simulink model "MotorControl_4"  (Simulink 8.1)
settings: Solver=FixedStepDiscrete  StartTime=0.0  StopTime=20  FixedStep=0.02  RelTol=1e-3
PostLoadFcn:
  | MotorControl_4_data
undefined symbols (not defined in the file or in its folder): A14, B, B13, D, L3, R10
libraries: BAMLIB564xL x12, rappid_564xl_ec_toolbox x1
settings Model: Creator=evarshavskaya  LastModifiedBy=evarshavskaya
settings DataIOCC: ExternalInput=off  InitialState=off  SaveOutput=off  SignalLogging=off  SaveTime=off
settings OptimizationCC: InlineParams=on  OptimizeModelRefInitCode=on  LifeSpan=1
settings DebuggingCC: InheritedTsInSrcMsg=none  SingleTaskRateTransMsg=error  ParameterPrecisionLossMsg=none  UnconnectedInputMsg=error  UnconnectedOutputMsg=error  UnconnectedLineMsg=error  UnknownTsInhSupMsg=error
settings HardwareCC: ProdLargestAtomicInteger=Long  ProdLargestAtomicFloat=Double  ProdIntDivRoundTo=Zero  ProdEndianess=BigEndian  ProdHWDeviceType=Freescale->32-bit PowerPC
settings RTWCC: SystemTargetFile=rappid564xl.tlc  MakeCommand=rappid_564xl_make_rtw  TemplateMakefile=rappid_564xl_default_tmf  PostCodeGenCommand=rappid_analyzegencode(buildInfo)  Description=RAppID Toolbox MPC564xL Code Generation Target (rappid)  ProcessScript=rappid564xl_make_rtw_hook
settings CodeAppCC: IgnoreCustomStorageClasses=off  CustomSymbolStrType=$N$R$M  InternalIdentifier=Classic
settings STFCustomTargetCC: CodeReplacementLibrary=ANSI_C  ModelReferenceCompliant=off  CombineOutputUpdateFcns=on  SuppressErrorStatus=on  ERTCustomFileBanners=on  SupportContinuousTime=off  SupportNonInlinedSFcns=off  MATLABClassNameForMDSCustomization=Simulink.SoftwareTarget.ERTCustomization  GRTInterface=off  SystemTargetFile=rappid564xl.tlc
settings ERTTargetCC: CodeReplacementLibrary=ANSI_C  MultiwordLength=2048  ModelReferenceCompliant=off  ParMdlRefBuildCompliant=off  CompOptLevelCompliant=off  ConcurrentExecutionCompliant=off  SuppressErrorStatus=on  ERTFirstTimeCompliant=off  ModelStepFunctionPrototypeControlCompliant=off  CPPClassGenCompliant=off  ExtModeMexFile=noextcomm  InlinedParameterPlacement=NonHierarchical  ERTCustomFileTemplate=example_file_process.tlc  ConvertIfToSwitch=off  SuppressUnreachableDefaultCases=off

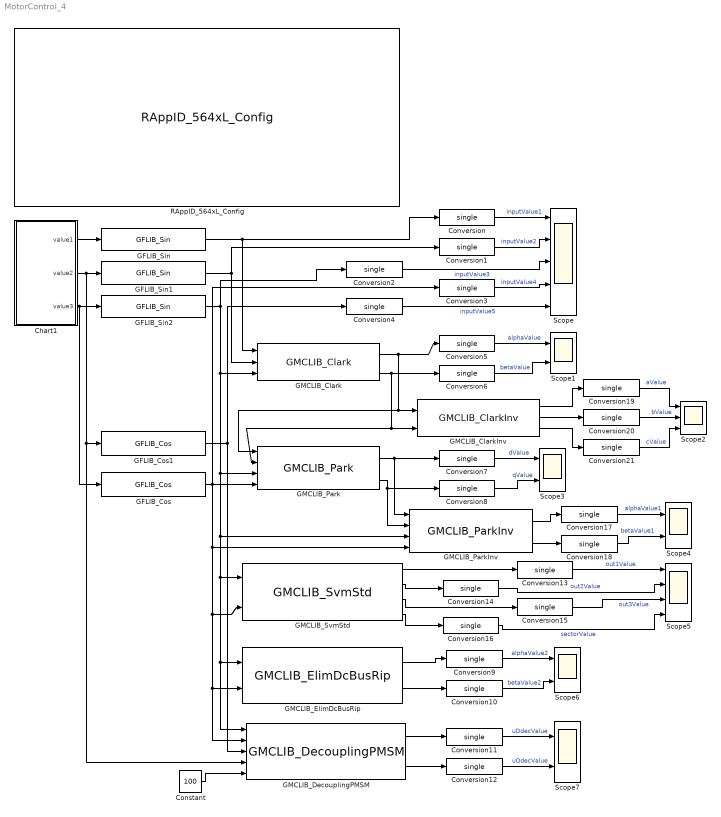
== system MotorControl_4 ==
  Chart1 : Stateflow chart  TreatAsAtomicUnit=on
  Constant : Constant  Value=100  OutDataTypeStr=single
  Conversion{,1..21} (22 alike) : DataTypeConversion  OutDataTypeStr=single
  GFLIB_Cos : BAMLIB564xL/General Functions/GFLIB_Cos
  GFLIB_Cos1 : BAMLIB564xL/General Functions/GFLIB_Cos
  GFLIB_Sin : BAMLIB564xL/General Functions/GFLIB_Sin
  GFLIB_Sin1 : BAMLIB564xL/General Functions/GFLIB_Sin
  GFLIB_Sin2 : BAMLIB564xL/General Functions/GFLIB_Sin
  GMCLIB_Clark : BAMLIB564xL/General Motor Control Functions/GMCLIB_Clark
  GMCLIB_ClarkInv : BAMLIB564xL/General Motor Control Functions/GMCLIB_ClarkInv
  GMCLIB_DecouplingPMSM : BAMLIB564xL/General Motor Control Functions/GMCLIB_DecouplingPMSM  s32Ld=s32Kd  s32Lq=s32Kq
  GMCLIB_ElimDcBusRip : BAMLIB564xL/General Motor Control Functions/GMCLIB_ElimDcBusRip  s32ModIndex=s32ModIndex  s32ArgDcBusMsr=s32ArgDcBusMsr
  GMCLIB_Park : BAMLIB564xL/General Motor Control Functions/GMCLIB_Park
  GMCLIB_ParkInv : BAMLIB564xL/General Motor Control Functions/GMCLIB_ParkInv
  GMCLIB_SvmStd : BAMLIB564xL/General Motor Control Functions/GMCLIB_SvmStd
  RAppID_564xL_Config : rappid_564xl_ec_toolbox/MPC564xL/RAppID_564xL_Config  SystemClock=120  XTAL=40  MC_clock_60=12  MC_clock_80=16  MC_clock_120=10  SWG_clock_60=20  SWG_clock_80=13.334  SWG_clock_120=20  Compiler=CodeWarrior  MemTarget=RAM  Part=MPC5643L  Package=144 LQFP  global_int_priority=10  base_tick_priority=14  sys_task_supress=off  exception_handlers=off  stored_mdl_name=MotorControl_4  freemaster_interface=Oops  freemaster_rx_pin="LINFlex_0 Rx Pin 116 : \"PB[3]\""  freemaster_tx_pin="LINFlex_0 Tx Pin 114 : \"PB[2]\""  freemaster_interface_1=Serial 0  freemaster_enable=on  freemaster_rate=57600  freemaster_tx0_pin=18 : B[2] : 114 : A14  freemaster_rx0_pin=19 : B[3] : 116 : B13  freemaster_tx1_pin=57 : D[9] : 26 : L3  freemaster_rx1_pin=29 : B[13] : 60 : R10  freemaster_can_channel=1CH  freemater_can_speed=500K  freemaster_can_msgig=0x7AA  ccp_interface=None  ccp_enable=off  ccp_can_channel=CH1 (MB 0 - 1)  ccp_can_speed=500K  ccp_can_cro_id=256  ccp_can_dto_id=257  ccp_dev_id=RappID  ccp_dev_addr=0  ccp_odt=3  ccp_daq=3  pil_enable=off  pil_bam=on  comport=1  pil_rate=57600  bam_password_def=on  bam_password=0xFEEDFACECAFEBEEF  bam_sa_cs=off  bam_start_address=0x0  bam_code_size=0x7000  cons_dspi=on  cons_can=on  cons_adc=on  cons_pwm=on  cons_ctu=on  cons_swg=on  cons_eTimer=on  cons_fm=on
  Scope : Scope  NumInputPorts=5
      settings: TickLabels=on  TimeRange=20  YMin=-1~-1~-1~-1~-1  YMax=1~1~1~1~1
  Scope{1,3..4,6..7} (5 alike) : Scope  NumInputPorts=2
      Scope1 settings: TickLabels=on  TimeRange=20  YMin=-1~-1  YMax=1~1
      Scope3 settings: TickLabels=on  TimeRange=20  YMin=-1.2~-1  YMax=0~1  SaveName=ScopeData3
      Scope4 settings: TickLabels=on  TimeRange=20  YMin=-1~-1  YMax=1~1  SaveName=ScopeData4
      Scope6 settings: TickLabels=on  TimeRange=20  YMin=-1~-1  YMax=1~1  SaveName=ScopeData6
      Scope7 settings: TickLabels=on  TimeRange=20  YMin=-10~-8  YMax=5~8  SaveName=ScopeData7
  Scope2 : Scope  NumInputPorts=3
      settings: TickLabels=on  TimeRange=20  YMin=-1~-1~-1  YMax=1~1~1  SaveName=ScopeData2
  Scope5 : Scope  NumInputPorts=4
      settings: TickLabels=on  TimeRange=20  YMin=-1~-1~-1~1  YMax=1~1~1~6  SaveName=ScopeData5
  wires:
  Chart1/1(value1) -> GFLIB_Sin/1
  GFLIB_Sin/1 -> GMCLIB_Clark/1, Conversion/1
  Chart1/2(value2) -> GFLIB_Sin1/1, GFLIB_Cos1/1, GMCLIB_DecouplingPMSM/4
  Chart1/3(value3) -> GFLIB_Sin2/1, GFLIB_Cos/1
  GFLIB_Sin1/1 -> GMCLIB_Clark/2, Conversion1/1
  GFLIB_Sin2/1 -> GMCLIB_Clark/3, GMCLIB_Park/3, GMCLIB_ParkInv/3, GMCLIB_SvmStd/1, GMCLIB_ElimDcBusRip/1, GMCLIB_DecouplingPMSM/1, Conversion2/1
  GMCLIB_Clark/1 -> GMCLIB_Park/1, GMCLIB_ClarkInv/1, Conversion5/1
  GMCLIB_Clark/2 -> GMCLIB_ClarkInv/2, GMCLIB_Park/2, Conversion6/1
  GMCLIB_ClarkInv/1 -> Conversion19/1
  GMCLIB_ClarkInv/2 -> Conversion20/1
  GMCLIB_ClarkInv/3 -> Conversion21/1
  GFLIB_Cos/1 -> GMCLIB_Park/4, GMCLIB_ParkInv/4, GMCLIB_SvmStd/2, GMCLIB_ElimDcBusRip/2, GMCLIB_DecouplingPMSM/2, Conversion3/1
  GMCLIB_Park/1 -> GMCLIB_ParkInv/1, Conversion7/1
  GMCLIB_Park/2 -> GMCLIB_ParkInv/2, Conversion8/1
  GMCLIB_ParkInv/1 -> Conversion17/1
  GMCLIB_ParkInv/2 -> Conversion18/1
  GMCLIB_SvmStd/1 -> Conversion13/1
  GMCLIB_SvmStd/2 -> Conversion14/1
  GMCLIB_SvmStd/3 -> Conversion15/1
  GMCLIB_SvmStd/4 -> Conversion16/1
  GMCLIB_ElimDcBusRip/1 -> Conversion9/1
  GMCLIB_ElimDcBusRip/2 -> Conversion10/1
  GFLIB_Cos1/1 -> GMCLIB_DecouplingPMSM/3, Conversion4/1
  Constant/1 -> GMCLIB_DecouplingPMSM/5
  GMCLIB_DecouplingPMSM/1 -> Conversion11/1
  GMCLIB_DecouplingPMSM/2 -> Conversion12/1
  Conversion/1 -> Scope/1  "inputValue1"
  Conversion1/1 -> Scope/2  "inputValue2"
  Conversion2/1 -> Scope/3  "inputValue3"
  Conversion3/1 -> Scope/4  "inputValue4"
  Conversion4/1 -> Scope/5  "inputValue5"
  Conversion5/1 -> Scope1/1  "alphaValue"
  Conversion6/1 -> Scope1/2  "betaValue"
  Conversion7/1 -> Scope3/1  "dValue"
  Conversion8/1 -> Scope3/2  "qValue"
  Conversion9/1 -> Scope6/1  "alphaValue2"
  Conversion10/1 -> Scope6/2  "betaValue2"
  Conversion11/1 -> Scope7/1  "uDdecValue"
  Conversion12/1 -> Scope7/2  "uQdecValue"
  Conversion13/1 -> Scope5/1  "out1Value"
  Conversion14/1 -> Scope5/2  "out2Value"
  Conversion15/1 -> Scope5/3  "out3Value"
  Conversion16/1 -> Scope5/4  "sectorValue"
  Conversion17/1 -> Scope4/1  "alphaValue1"
  Conversion18/1 -> Scope4/2  "betaValue1"
  Conversion20/1 -> Scope2/2  "bValue"
  Conversion19/1 -> Scope2/1  "aValue"
  Conversion21/1 -> Scope2/3  "cValue"

== stateflow chart Chart1 ==
  settings: executeAtInitialization=1
  state A
    du:
    cntr=cntr+0.02;
    value1=cntr;
    value2=value1+1;
    value3=value2+1;
    ex:
    cntr = -3.14;
  (default) -> A : {cntr=0;}
  A -> A : [cntr >= 3.14]
  data: cntr local single [-4..4] =0; value1 output single [-4..4]; value2 output single [-3..5]; value3 output single [-2..6]
